simulink model "dcac_switching"  (Simulink 6.5)
settings: Solver=ode45  StartTime=0.0  StopTime=1/60  MaxStep=0.1e-6  RelTol=1e-3
settings Model: Creator=Mama  LastModifiedBy=Dragan Maksimovic
settings DebuggingCC: AlgebraicLoopMsg=none  SolverPrmCheckMsg=none  UnconnectedOutputMsg=none

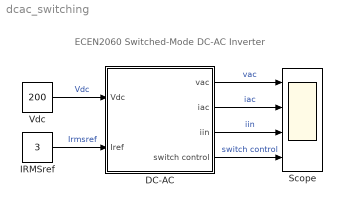
== system dcac_switching ==
  note: ECEN2060
      | Switched-Mode DC-AC Inverter
  DC-AC : Subsystem  mask{Vrms=120, f=60, L=2e-3, DeltaI=1}
      mask prompts: Vrms "AC line RMS voltage"; f "AC line frequency"; L "Inductance"; DeltaI "Inductor current ripple"
      mask help: Switched-mode DC-AC inverter for single-phase grid-connected systems. Output current, which is controlled using a comparator with hysteresis, is in phase with the AC line voltage and has the RMS value set by an input reference. The model is ideal, losses are neglected, efficiency is 100%
      mask Display:
      | text(0.5,0.75,'DC-AC','horizontalAlignment', 'center');
      | text(0.5,0.6,'inverter','horizontalAlignment', 'center');
      | text(0.5,0.45,'(switching)','horizontalAlignment', 'center');
  IRMSref : Constant  Value=3  OutDataType=sfix(16)  ConRadixGroup=Use specified scaling  OutScaling=2^0  SampleTime=inf  FramePeriod=inf
  Scope : Scope  NumInputPorts=4
      settings: TimeRange=0.018  YMin=-200~-5~-5~-0.5  YMax=200~5~5~1.5
  Vdc : Constant  Value=200  OutDataType=sfix(16)  ConRadixGroup=Use specified scaling  OutScaling=2^0  SampleTime=inf  FramePeriod=inf
  wires:
  Vdc/1 -> DC-AC/1(Vdc)  "Vdc"
  IRMSref/1 -> DC-AC/2(Iref)  "Irmsref"
  DC-AC/1(vac) -> Scope/1  "vac"
  DC-AC/2(iac) -> Scope/2  "iac"
  DC-AC/3(iin) -> Scope/3  "iin"
  DC-AC/4(switch control) -> Scope/4  "switch control"

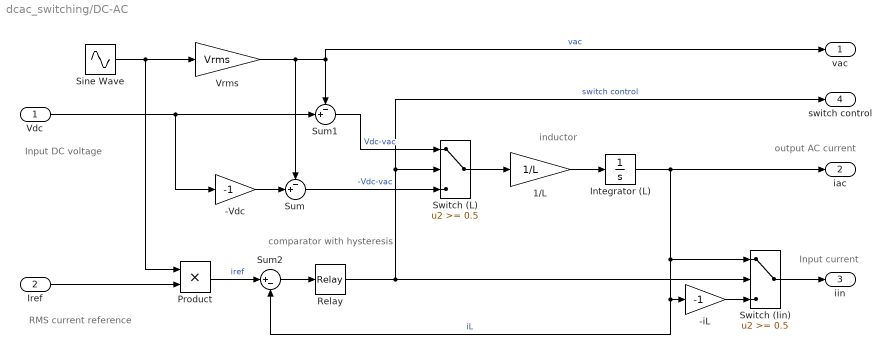
== system dcac_switching/DC-AC ==
  note: output AC current
  note: Input current
  note: Input DC voltage
  note: RMS current reference
  note: inductor
  note: comparator
      | with hysteresis
  Vdc : Inport
  Iref : Inport  Port=2
  -Vdc : Gain  Gain=-1
  -iL : Gain  Gain=-1
  1/L : Gain  Gain=1/L
  Integrator (L) : Integrator  InitialCondition=4
  Product : Product  RndMeth=Zero
  Relay : Relay  OnSwitchValue=DeltaI/2  OffSwitchValue=-DeltaI/2
  Sine Wave : Sin  Amplitude=1*sqrt(2)  Frequency=2*pi*f  SampleTime=0
  Sum : Sum  Inputs=-+|
  Sum1 : Sum  Inputs=-+|
  Sum2 : Sum  Inputs=|+-
  Switch (Iin) : Switch  Threshold=0.5
  Switch (L) : Switch  Threshold=0.5
  Vrms : Gain  Gain=Vrms
  vac : Outport
  iac : Outport  Port=2
  iin : Outport  Port=3
  switch control : Outport  Port=4
  wires:
  Vdc/1 -> -Vdc/1, Sum1/2
  Switch (L)/1 -> 1/L/1
  1/L/1 -> Integrator (L)/1
  Integrator (L)/1 -> Switch (Iin)/1, -iL/1, Sum2/2, iac/1  "iL"
  -Vdc/1 -> Sum/2
  Sum/1 -> Switch (L)/3  "-Vdc-vac"
  Sum1/1 -> Switch (L)/1  "Vdc-vac"
  Sine Wave/1 -> Vrms/1, Product/1
  Vrms/1 -> Sum/1, Sum1/1, vac/1  "vac"
  -iL/1 -> Switch (Iin)/3
  Product/1 -> Sum2/1  "iref"
  Iref/1 -> Product/2
  Sum2/1 -> Relay/1
  Relay/1 -> Switch (Iin)/2, Switch (L)/2, switch control/1  "switch control"
  Switch (Iin)/1 -> iin/1
